simulink model "verify_sfun_storage_heatexchanger_mdl"  (R2018b)
settings: Solver=VariableStepDiscrete  StartTime=0.0  StopTime=1  MaxStep=1  RelTol=1e-3  EnableMultiTasking=on
libraries: carnot x5
settings Model: Creator=drhf  LastModifiedBy=drhf
settings DataIOCC: LimitDataPoints=on  SaveFormat=Array  SignalLoggingSaveFormat=ModelDataLogs
settings OptimizationCC: ExpressionDepthLimit=2147483647  LifeSpan=inf
settings DebuggingCC: UnderspecifiedInitializationDetection=Classic  MergeDetectMultiDrivingBlocksExec=none  SolverPrmCheckMsg=warning  FcnCallInpInsideContextMsg=warning  StateNameClashWarn=warning  SFUnexpectedBacktrackingDiag=warning  SFNoUnconditionalDefaultTransitionDiag=warning  SFExecutionAtInitializationDiag=none
settings HardwareCC: ProdBitPerPointer=32  ProdBitPerSizeT=32  ProdBitPerPtrDiffT=32  ProdLargestAtomicFloat=None  ProdIntDivRoundTo=Undefined  ProdEndianess=Unspecified  ProdWordSize=32  ProdHWDeviceType=32-bit Generic
settings ModelReferenceCC: PropagateSignalLabelsOutOfModel=off
settings SFSimCC: SimUseLocalCustomCode=off
settings RTWCC: RTWUseLocalCustomCode=off
settings CodeAppCC: StateflowObjectComments=on
settings GRTTargetCC: TargetLangStandard=C89/C90 (ANSI)  GeneratePreprocessorConditionals=Disable all  CombineOutputUpdateFcns=off  GRTInterface=on
settings ConfigComp: CovMetricSettings=dw  CovHtmlReporting=on  CovSaveCumulativeToWorkspaceVar=on  CovSaveSingleToWorkspaceVar=on  CovExternalEMLEnable=off

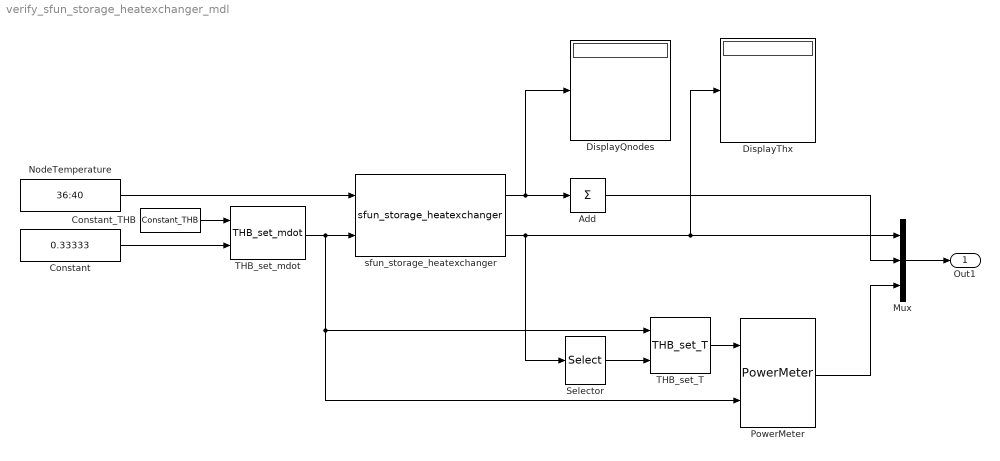
== system verify_sfun_storage_heatexchanger_mdl ==
  Add : Sum  Inputs=1
  Constant : Constant  Value=0.33333
  Constant_THB : carnot/Source/Simple/Constant_THB  t=40  mdot=1/3600  p=1e5  mID=No Pressure Drop  fluid=Water  mix=0  mix2=0  mix3=0  dia=0.02  hgt=0
      settings: SourceProductName=Carnot
  DisplayQnodes : Display
  DisplayThx : Display
  Mux : Mux  Inputs=3
  NodeTemperature : Constant  Value=36:40
  PowerMeter : carnot/Control/PowerMeter
      settings: SourceProductName=Carnot
  Selector : Selector  InputPortWidth=5  IndexOptions=Index vector (dialog)  Indices=1  OutputSizes=1
  THB_set_T : carnot/Source/Simple/THB_set_T
      settings: SourceProductName=Carnot
  THB_set_mdot : carnot/Source/Simple/THB_set_mdot
      settings: SourceProductName=Carnot
  sfun_storage_heatexchanger : carnot/Basic/Thermal_Models/sfun_storage_heatexchanger  idn=heat transfer from data fit  nodes=5  inlet=5  outlet=1  p1=100  p2=0  p3=0  p4=0  p5=0  p6=0  p7=0
      settings: SourceProductName=Carnot
  Out1 : Outport
  wires:
  NodeTemperature/1 -> sfun_storage_heatexchanger/1
  sfun_storage_heatexchanger/1 -> DisplayQnodes/1, Add/1
  sfun_storage_heatexchanger/2 -> DisplayThx/1, Mux/1, Selector/1
  Constant_THB/1 -> THB_set_mdot/1
  THB_set_mdot/1 -> sfun_storage_heatexchanger/2, THB_set_T/1, PowerMeter/2
  Constant/1 -> THB_set_mdot/2
  Mux/1 -> Out1/1
  THB_set_T/1 -> PowerMeter/1
  PowerMeter/1 -> Mux/3
  Add/1 -> Mux/2
  Selector/1 -> THB_set_T/2
